simulink model "GS_model"  (R2018b)
settings: Solver=ode5  StartTime=0.0  StopTime=SimuStopTime  FixedStep=T_Simu  RelTol=1e-3
InitFcn:
  | Initial
undefined symbols (not defined in the file or in its folder): Aba10, Aba20, aeroCIP2006_S, aeroCIP2006_X, aeroCIP2006_Y, Agl0, Ass_kS, Ass_n1, Ass_n2, Ass_n3, Ass_n4, Ass_Noise, Ass_R, Ass_Resolution, Ass_TmOrder, AssA_Fix_Abs, AssB_Fix_Abs, AssC_Fix_Abs, AssD_Fix_Abs, AssE_Fix_Aps, AssF_Fix_Aps, C, c_max, c_min, Cd, CenterOfFigNX, CenterOfFigNY, CenterOfFigNZ, CenterOfFigP1, CenterOfFigP2, CenterOfFigPX, CenterOfFigPY, CenterOfFigPZ, Cmu, Crou, DEG2RAD, DiscIntNeverNeededParam, Eg_Dir, Eg_F, Eg_PrepareTime, Eg_r_L_L, Fw_Abf, Fw_Hmax, Fw_J, Fw_Spd0, Fw_Tmax, git_hash_BaseLine, git_hash_Project, Gnss_Noise_Pos, Gnss_Noise_Vel, Gnss_PropgationTime, GyroA_Fix_Abg, GyroA_Noise, GyroB_Fix_Abg, GyroB_Noise, GyroC_Fix_Abg, GyroC_Noise, GyroD_Fix_Abg, GyroD_Noise, h ... (+94)
libraries: simulink x308, sharedutil x46, aerolibutil x37, sharedtransform x31, vrlib x14, aerolibgravity2 x2
(part 13 of 20)

== system GS_model/Subsystem2/Subsystem/Sensor/StA&B&C&DModel1/StAMathModel3/Subsystem/Subsystem ==
  note: Qbs
  Sun_b : Inport
  Sunshine : Inport  Port=2
  Qsb_StAFix : Inport  Port=3
  SEA : Inport  Port=4
  EEA : Inport  Port=5
  Qob : Inport  Port=6
  Acos : Trigonometry  Operator=acos
  Acos1 : Trigonometry  Operator=acos
  Compare To Constant : simulink/Logic and Bit Operations/Compare To Constant  relop===  const=1  OutDataTypeStr=boolean
  Constant : Constant  Value=St_SightAxis
  Constant1 : Constant  Value=[0;0;1]
  Constant3 : Constant  Value=St_EarthAtomAgl
  Cos : Trigonometry  Operator=cos
  Cos1 : Trigonometry  Operator=cos
  Data Type Conversion : DataTypeConversion  OutDataTypeStr=double
  Logical Operator : Logic  AllPortsSameDT=off  OutDataTypeStr=boolean
  Logical Operator1 : Logic  Operator=OR  AllPortsSameDT=off  OutDataTypeStr=boolean
  Logical Operator2 : Logic  Operator=NOT  AllPortsSameDT=off  OutDataTypeStr=boolean
  MatrixMultiply{,1..4} (5 alike) : Product  Multiplication=Matrix(*)
  Mux : Mux  Inputs=2
  Quaternion Inverse : aerolibutil/Quaternion Inverse
  Quaternions to Direction Cosine Matrix : sharedtransform/Quaternions to  Direction Cosine Matrix  aMode=aMode
      settings: SourceProductBaseCode=AE,PW,MT,VE,VP
  Quaternions to Direction Cosine Matrix1 : sharedtransform/Quaternions to  Direction Cosine Matrix  aMode=aMode
      settings: SourceProductBaseCode=AE,PW,MT,VE,VP
  Relational Operator : RelationalOperator  OutDataTypeStr=boolean  RndMeth=Simplest
  Relational Operator1 : RelationalOperator  OutDataTypeStr=boolean  RndMeth=Simplest
  Sum : Sum  Inputs=|++
  Transpose : Math  Operator=transpose  SaturateOnIntegerOverflow=on
  Valid : Outport
  Agl_St&SunEarth : Outport  Port=2
  wires:
  Logical Operator1/1 -> Logical Operator2/1
  Data Type Conversion/1 -> Valid/1
  Logical Operator2/1 -> Data Type Conversion/1
  Mux/1 -> Agl_St&SunEarth/1
  MatrixMultiply/1 -> MatrixMultiply1/2
  Compare To Constant/1 -> Logical Operator/1
  MatrixMultiply1/1 -> Acos/1, Relational Operator/1
  Sum/1 -> Cos1/1
  Acos1/1 -> Mux/2
  Acos/1 -> Mux/1
  Relational Operator1/1 -> Logical Operator1/2
  EEA/1 -> Sum/1
  Sunshine/1 -> Compare To Constant/1
  MatrixMultiply4/1 -> Relational Operator1/1, Acos1/1
  Constant/1 -> Transpose/1
  Relational Operator/1 -> Logical Operator/2
  Quaternion Inverse/1 -> Quaternions to Direction Cosine Matrix/1
  Cos1/1 -> Relational Operator1/2
  MatrixMultiply2/1 -> MatrixMultiply3/2
  Constant1/1 -> MatrixMultiply2/2
  Sun_b/1 -> MatrixMultiply/2
  Quaternions to Direction Cosine Matrix/1 -> MatrixMultiply/1, MatrixMultiply3/1
  Qsb_StAFix/1 -> Quaternion Inverse/1
  MatrixMultiply3/1 -> MatrixMultiply4/2
  Qob/1 -> Quaternions to Direction Cosine Matrix1/1
  SEA/1 -> Cos/1
  Quaternions to Direction Cosine Matrix1/1 -> MatrixMultiply2/1
  Cos/1 -> Relational Operator/2
  Logical Operator/1 -> Logical Operator1/1
  Constant3/1 -> Sum/2
  Transpose/1 -> MatrixMultiply1/1, MatrixMultiply4/1

== system GS_model/Subsystem2/Subsystem/Sensor/StA&B&C&DModel1/StAMathModel3/Subsystem/Triggered Subsystem2 ==
  In1 : Inport
  Enable : EnablePort
  Out1 : Outport  InitialOutput=1
  wires:
  In1/1 -> Out1/1

== system GS_model/Subsystem2/EquipmentCmd/Fw1/Subsystem7/Subsystem1/FWDataSourceChoice/CmdModeChoice/422 ==
  In1 : Inport
  Action Port : ActionPort  ActionType=then
  Out1 : Outport
  wires:
  In1/1 -> Out1/1

== system GS_model/Subsystem2/EquipmentCmd/Fw1/Subsystem7/Subsystem1/FWDataSourceChoice/CmdModeChoice/FC ==
  In1 : Inport
  Action Port : ActionPort  ActionType=else
  Out1 : Outport
  wires:
  In1/1 -> Out1/1

== system GS_model/Subsystem2/EquipmentCmd/Fw1/Subsystem7/Subsystem1/FWDataSourceChoice/CmdModeChoice/UDP ==
  In1 : Inport
  Action Port : ActionPort  ActionType=elseif
  Out1 : Outport
  wires:
  In1/1 -> Out1/1

== system GS_model/Subsystem2/EquipmentCmd/Fw1/Subsystem7/Subsystem1/FWDataSourceChoice/CmdSpdChoice/422 ==
  In1 : Inport
  Action Port : ActionPort  ActionType=then
  Out1 : Outport
  wires:
  In1/1 -> Out1/1

== system GS_model/Subsystem2/EquipmentCmd/Fw1/Subsystem7/Subsystem1/FWDataSourceChoice/CmdSpdChoice/FC ==
  In1 : Inport
  Action Port : ActionPort  ActionType=else
  Out1 : Outport
  wires:
  In1/1 -> Out1/1

== system GS_model/Subsystem2/EquipmentCmd/Fw1/Subsystem7/Subsystem1/FWDataSourceChoice/CmdSpdChoice/UDP ==
  In1 : Inport
  Action Port : ActionPort  ActionType=elseif
  Out1 : Outport
  wires:
  In1/1 -> Out1/1

== system GS_model/Subsystem2/EquipmentCmd/Fw1/Subsystem7/Subsystem1/FWDataSourceChoice/CmdTChoice/422 ==
  In1 : Inport
  Action Port : ActionPort  ActionType=then
  Out1 : Outport
  wires:
  In1/1 -> Out1/1

== system GS_model/Subsystem2/EquipmentCmd/Fw1/Subsystem7/Subsystem1/FWDataSourceChoice/CmdTChoice/FC ==
  In1 : Inport
  Action Port : ActionPort  ActionType=else
  Out1 : Outport
  wires:
  In1/1 -> Out1/1

== system GS_model/Subsystem2/EquipmentCmd/Fw1/Subsystem7/Subsystem1/FWDataSourceChoice/CmdTChoice/UDP ==
  In1 : Inport
  Action Port : ActionPort  ActionType=elseif
  Out1 : Outport
  wires:
  In1/1 -> Out1/1

== system GS_model/Subsystem2/EquipmentCmd/Fw1/Subsystem7/Subsystem2/FWDataSourceChoice/CmdModeChoice/422 ==
  In1 : Inport
  Action Port : ActionPort  ActionType=then
  Out1 : Outport
  wires:
  In1/1 -> Out1/1

== system GS_model/Subsystem2/EquipmentCmd/Fw1/Subsystem7/Subsystem2/FWDataSourceChoice/CmdModeChoice/FC ==
  In1 : Inport
  Action Port : ActionPort  ActionType=else
  Out1 : Outport
  wires:
  In1/1 -> Out1/1

== system GS_model/Subsystem2/EquipmentCmd/Fw1/Subsystem7/Subsystem2/FWDataSourceChoice/CmdModeChoice/UDP ==
  In1 : Inport
  Action Port : ActionPort  ActionType=elseif
  Out1 : Outport
  wires:
  In1/1 -> Out1/1

== system GS_model/Subsystem2/EquipmentCmd/Fw1/Subsystem7/Subsystem2/FWDataSourceChoice/CmdSpdChoice/422 ==
  In1 : Inport
  Action Port : ActionPort  ActionType=then
  Out1 : Outport
  wires:
  In1/1 -> Out1/1

== system GS_model/Subsystem2/EquipmentCmd/Fw1/Subsystem7/Subsystem2/FWDataSourceChoice/CmdSpdChoice/FC ==
  In1 : Inport
  Action Port : ActionPort  ActionType=else
  Out1 : Outport
  wires:
  In1/1 -> Out1/1

== system GS_model/Subsystem2/EquipmentCmd/Fw1/Subsystem7/Subsystem2/FWDataSourceChoice/CmdSpdChoice/UDP ==
  In1 : Inport
  Action Port : ActionPort  ActionType=elseif
  Out1 : Outport
  wires:
  In1/1 -> Out1/1

== system GS_model/Subsystem2/EquipmentCmd/Fw1/Subsystem7/Subsystem2/FWDataSourceChoice/CmdTChoice/422 ==
  In1 : Inport
  Action Port : ActionPort  ActionType=then
  Out1 : Outport
  wires:
  In1/1 -> Out1/1

== system GS_model/Subsystem2/EquipmentCmd/Fw1/Subsystem7/Subsystem2/FWDataSourceChoice/CmdTChoice/FC ==
  In1 : Inport
  Action Port : ActionPort  ActionType=else
  Out1 : Outport
  wires:
  In1/1 -> Out1/1

== system GS_model/Subsystem2/EquipmentCmd/Fw1/Subsystem7/Subsystem2/FWDataSourceChoice/CmdTChoice/UDP ==
  In1 : Inport
  Action Port : ActionPort  ActionType=elseif
  Out1 : Outport
  wires:
  In1/1 -> Out1/1

== system GS_model/Subsystem2/EquipmentCmd/Fw1/Subsystem7/Subsystem3/FWDataSourceChoice/CmdModeChoice/422 ==
  In1 : Inport
  Action Port : ActionPort  ActionType=then
  Out1 : Outport
  wires:
  In1/1 -> Out1/1

== system GS_model/Subsystem2/EquipmentCmd/Fw1/Subsystem7/Subsystem3/FWDataSourceChoice/CmdModeChoice/FC ==
  In1 : Inport
  Action Port : ActionPort  ActionType=else
  Out1 : Outport
  wires:
  In1/1 -> Out1/1

== system GS_model/Subsystem2/EquipmentCmd/Fw1/Subsystem7/Subsystem3/FWDataSourceChoice/CmdModeChoice/UDP ==
  In1 : Inport
  Action Port : ActionPort  ActionType=elseif
  Out1 : Outport
  wires:
  In1/1 -> Out1/1

== system GS_model/Subsystem2/EquipmentCmd/Fw1/Subsystem7/Subsystem3/FWDataSourceChoice/CmdSpdChoice/422 ==
  In1 : Inport
  Action Port : ActionPort  ActionType=then
  Out1 : Outport
  wires:
  In1/1 -> Out1/1

== system GS_model/Subsystem2/EquipmentCmd/Fw1/Subsystem7/Subsystem3/FWDataSourceChoice/CmdSpdChoice/FC ==
  In1 : Inport
  Action Port : ActionPort  ActionType=else
  Out1 : Outport
  wires:
  In1/1 -> Out1/1

== system GS_model/Subsystem2/EquipmentCmd/Fw1/Subsystem7/Subsystem3/FWDataSourceChoice/CmdSpdChoice/UDP ==
  In1 : Inport
  Action Port : ActionPort  ActionType=elseif
  Out1 : Outport
  wires:
  In1/1 -> Out1/1

== system GS_model/Subsystem2/EquipmentCmd/Fw1/Subsystem7/Subsystem3/FWDataSourceChoice/CmdTChoice/422 ==
  In1 : Inport
  Action Port : ActionPort  ActionType=then
  Out1 : Outport
  wires:
  In1/1 -> Out1/1

== system GS_model/Subsystem2/EquipmentCmd/Fw1/Subsystem7/Subsystem3/FWDataSourceChoice/CmdTChoice/FC ==
  In1 : Inport
  Action Port : ActionPort  ActionType=else
  Out1 : Outport
  wires:
  In1/1 -> Out1/1

== system GS_model/Subsystem2/EquipmentCmd/Fw1/Subsystem7/Subsystem3/FWDataSourceChoice/CmdTChoice/UDP ==
  In1 : Inport
  Action Port : ActionPort  ActionType=elseif
  Out1 : Outport
  wires:
  In1/1 -> Out1/1

== system GS_model/Subsystem2/EquipmentCmd/Fw1/Subsystem7/Subsystem4/FWDataSourceChoice/CmdModeChoice/422 ==
  In1 : Inport
  Action Port : ActionPort  ActionType=then
  Out1 : Outport
  wires:
  In1/1 -> Out1/1

== system GS_model/Subsystem2/EquipmentCmd/Fw1/Subsystem7/Subsystem4/FWDataSourceChoice/CmdModeChoice/FC ==
  In1 : Inport
  Action Port : ActionPort  ActionType=else
  Out1 : Outport
  wires:
  In1/1 -> Out1/1

== system GS_model/Subsystem2/EquipmentCmd/Fw1/Subsystem7/Subsystem4/FWDataSourceChoice/CmdModeChoice/UDP ==
  In1 : Inport
  Action Port : ActionPort  ActionType=elseif
  Out1 : Outport
  wires:
  In1/1 -> Out1/1

== system GS_model/Subsystem2/EquipmentCmd/Fw1/Subsystem7/Subsystem4/FWDataSourceChoice/CmdSpdChoice/422 ==
  In1 : Inport
  Action Port : ActionPort  ActionType=then
  Out1 : Outport
  wires:
  In1/1 -> Out1/1

== system GS_model/Subsystem2/EquipmentCmd/Fw1/Subsystem7/Subsystem4/FWDataSourceChoice/CmdSpdChoice/FC ==
  In1 : Inport
  Action Port : ActionPort  ActionType=else
  Out1 : Outport
  wires:
  In1/1 -> Out1/1

== system GS_model/Subsystem2/EquipmentCmd/Fw1/Subsystem7/Subsystem4/FWDataSourceChoice/CmdSpdChoice/UDP ==
  In1 : Inport
  Action Port : ActionPort  ActionType=elseif
  Out1 : Outport
  wires:
  In1/1 -> Out1/1

== system GS_model/Subsystem2/EquipmentCmd/Fw1/Subsystem7/Subsystem4/FWDataSourceChoice/CmdTChoice/422 ==
  In1 : Inport
  Action Port : ActionPort  ActionType=then
  Out1 : Outport
  wires:
  In1/1 -> Out1/1

== system GS_model/Subsystem2/EquipmentCmd/Fw1/Subsystem7/Subsystem4/FWDataSourceChoice/CmdTChoice/FC ==
  In1 : Inport
  Action Port : ActionPort  ActionType=else
  Out1 : Outport
  wires:
  In1/1 -> Out1/1

== system GS_model/Subsystem2/EquipmentCmd/Fw1/Subsystem7/Subsystem4/FWDataSourceChoice/CmdTChoice/UDP ==
  In1 : Inport
  Action Port : ActionPort  ActionType=elseif
  Out1 : Outport
  wires:
  In1/1 -> Out1/1

== system GS_model/Subsystem2/EquipmentCmd/Fw1/Subsystem7/Subsystem5/FWDataSourceChoice/CmdModeChoice/422 ==
  In1 : Inport
  Action Port : ActionPort  ActionType=then
  Out1 : Outport
  wires:
  In1/1 -> Out1/1

== system GS_model/Subsystem2/EquipmentCmd/Fw1/Subsystem7/Subsystem5/FWDataSourceChoice/CmdModeChoice/FC ==
  In1 : Inport
  Action Port : ActionPort  ActionType=else
  Out1 : Outport
  wires:
  In1/1 -> Out1/1

== system GS_model/Subsystem2/EquipmentCmd/Fw1/Subsystem7/Subsystem5/FWDataSourceChoice/CmdModeChoice/UDP ==
  In1 : Inport
  Action Port : ActionPort  ActionType=elseif
  Out1 : Outport
  wires:
  In1/1 -> Out1/1

== system GS_model/Subsystem2/EquipmentCmd/Fw1/Subsystem7/Subsystem5/FWDataSourceChoice/CmdSpdChoice/422 ==
  In1 : Inport
  Action Port : ActionPort  ActionType=then
  Out1 : Outport
  wires:
  In1/1 -> Out1/1

== system GS_model/Subsystem2/EquipmentCmd/Fw1/Subsystem7/Subsystem5/FWDataSourceChoice/CmdSpdChoice/FC ==
  In1 : Inport
  Action Port : ActionPort  ActionType=else
  Out1 : Outport
  wires:
  In1/1 -> Out1/1

== system GS_model/Subsystem2/EquipmentCmd/Fw1/Subsystem7/Subsystem5/FWDataSourceChoice/CmdSpdChoice/UDP ==
  In1 : Inport
  Action Port : ActionPort  ActionType=elseif
  Out1 : Outport
  wires:
  In1/1 -> Out1/1

== system GS_model/Subsystem2/EquipmentCmd/Fw1/Subsystem7/Subsystem5/FWDataSourceChoice/CmdTChoice/422 ==
  In1 : Inport
  Action Port : ActionPort  ActionType=then
  Out1 : Outport
  wires:
  In1/1 -> Out1/1

== system GS_model/Subsystem2/EquipmentCmd/Fw1/Subsystem7/Subsystem5/FWDataSourceChoice/CmdTChoice/FC ==
  In1 : Inport
  Action Port : ActionPort  ActionType=else
  Out1 : Outport
  wires:
  In1/1 -> Out1/1

== system GS_model/Subsystem2/EquipmentCmd/Fw1/Subsystem7/Subsystem5/FWDataSourceChoice/CmdTChoice/UDP ==
  In1 : Inport
  Action Port : ActionPort  ActionType=elseif
  Out1 : Outport
  wires:
  In1/1 -> Out1/1

== system GS_model/Subsystem2/EquipmentCmd/Fw1/Subsystem7/Subsystem6/FWDataSourceChoice/CmdModeChoice/422 ==
  In1 : Inport
  Action Port : ActionPort  ActionType=then
  Out1 : Outport
  wires:
  In1/1 -> Out1/1

== system GS_model/Subsystem2/EquipmentCmd/Fw1/Subsystem7/Subsystem6/FWDataSourceChoice/CmdModeChoice/FC ==
  In1 : Inport
  Action Port : ActionPort  ActionType=else
  Out1 : Outport
  wires:
  In1/1 -> Out1/1

== system GS_model/Subsystem2/EquipmentCmd/Fw1/Subsystem7/Subsystem6/FWDataSourceChoice/CmdModeChoice/UDP ==
  In1 : Inport
  Action Port : ActionPort  ActionType=elseif
  Out1 : Outport
  wires:
  In1/1 -> Out1/1

== system GS_model/Subsystem2/EquipmentCmd/Fw1/Subsystem7/Subsystem6/FWDataSourceChoice/CmdSpdChoice/422 ==
  In1 : Inport
  Action Port : ActionPort  ActionType=then
  Out1 : Outport
  wires:
  In1/1 -> Out1/1

== system GS_model/Subsystem2/EquipmentCmd/Fw1/Subsystem7/Subsystem6/FWDataSourceChoice/CmdSpdChoice/FC ==
  In1 : Inport
  Action Port : ActionPort  ActionType=else
  Out1 : Outport
  wires:
  In1/1 -> Out1/1

== system GS_model/Subsystem2/EquipmentCmd/Fw1/Subsystem7/Subsystem6/FWDataSourceChoice/CmdSpdChoice/UDP ==
  In1 : Inport
  Action Port : ActionPort  ActionType=elseif
  Out1 : Outport
  wires:
  In1/1 -> Out1/1

== system GS_model/Subsystem2/EquipmentCmd/Fw1/Subsystem7/Subsystem6/FWDataSourceChoice/CmdTChoice/422 ==
  In1 : Inport
  Action Port : ActionPort  ActionType=then
  Out1 : Outport
  wires:
  In1/1 -> Out1/1

== system GS_model/Subsystem2/EquipmentCmd/Fw1/Subsystem7/Subsystem6/FWDataSourceChoice/CmdTChoice/FC ==
  In1 : Inport
  Action Port : ActionPort  ActionType=else
  Out1 : Outport
  wires:
  In1/1 -> Out1/1

== system GS_model/Subsystem2/EquipmentCmd/Fw1/Subsystem7/Subsystem6/FWDataSourceChoice/CmdTChoice/UDP ==
  In1 : Inport
  Action Port : ActionPort  ActionType=elseif
  Out1 : Outport
  wires:
  In1/1 -> Out1/1

== system GS_model/Subsystem2/Subsystem/Actuator/FlyWheel/FwAModel1/FWDataSourceChoice/DelayModel/delay1 ==
  In1 : Inport
  In2 : Inport  Port=2
  Delay : Delay  DelayLength=floor(T_Ctrl/T_Simu)
  Delay1 : Delay  DelayLength=2*floor(T_Ctrl/T_Simu)
  Delay2 : Delay  DelayLength=3*floor(T_Ctrl/T_Simu)
  Delay3 : Delay  DelayLength=4*floor(T_Ctrl/T_Simu)
  Multiport Switch : MultiPortSwitch  Inputs=5  SaturateOnIntegerOverflow=on
  Out1 : Outport
  wires:
  Delay1/1 -> Multiport Switch/4
  Delay2/1 -> Multiport Switch/5
  Delay3/1 -> Multiport Switch/6
  In1/1 -> Multiport Switch/1
  Multiport Switch/1 -> Out1/1
  In2/1 -> Multiport Switch/2, Delay1/1, Delay2/1, Delay3/1, Delay/1
  Delay/1 -> Multiport Switch/3

== system GS_model/Subsystem2/Subsystem/Actuator/FlyWheel/FwAModel1/FWDataSourceChoice/DelayModel/delay2 ==
  In1 : Inport
  In2 : Inport  Port=2
  Delay : Delay  DelayLength=floor(T_Ctrl/T_Simu)
  Delay1 : Delay  DelayLength=2*floor(T_Ctrl/T_Simu)
  Delay2 : Delay  DelayLength=3*floor(T_Ctrl/T_Simu)
  Delay3 : Delay  DelayLength=4*floor(T_Ctrl/T_Simu)
  Multiport Switch : MultiPortSwitch  Inputs=5  SaturateOnIntegerOverflow=on
  Out1 : Outport
  wires:
  Delay/1 -> Multiport Switch/3
  In2/1 -> Delay/1, Delay3/1, Delay2/1, Delay1/1, Multiport Switch/2
  Multiport Switch/1 -> Out1/1
  In1/1 -> Multiport Switch/1
  Delay3/1 -> Multiport Switch/6
  Delay2/1 -> Multiport Switch/5
  Delay1/1 -> Multiport Switch/4

== system GS_model/Subsystem2/Subsystem/Actuator/FlyWheel/FwAModel1/FWDataSourceChoice/DelayModel/delay3 ==
  In1 : Inport
  In2 : Inport  Port=2
  Delay : Delay  DelayLength=floor(T_Ctrl/T_Simu)
  Delay1 : Delay  DelayLength=2*floor(T_Ctrl/T_Simu)
  Delay2 : Delay  DelayLength=3*floor(T_Ctrl/T_Simu)
  Delay3 : Delay  DelayLength=4*floor(T_Ctrl/T_Simu)
  Multiport Switch : MultiPortSwitch  Inputs=5  SaturateOnIntegerOverflow=on
  Out1 : Outport
  wires:
  Delay1/1 -> Multiport Switch/4
  Delay2/1 -> Multiport Switch/5
  Delay3/1 -> Multiport Switch/6
  In1/1 -> Multiport Switch/1
  Multiport Switch/1 -> Out1/1
  In2/1 -> Multiport Switch/2, Delay1/1, Delay2/1, Delay3/1, Delay/1
  Delay/1 -> Multiport Switch/3

== system GS_model/Subsystem2/Subsystem/Actuator/FlyWheel/FwAModel1/FWMath&ErrModel/Subsystem1/If Action Subsystem ==
  In1 : Inport
  Action Port : ActionPort  ActionType=then
  Out1 : Outport
  wires:
  In1/1 -> Out1/1

== system GS_model/Subsystem2/Subsystem/Actuator/FlyWheel/FwAModel1/FWMath&ErrModel/Subsystem1/If Action Subsystem1 ==
  In1 : Inport
  Action Port : ActionPort  ActionType=else
  Out1 : Outport
  wires:
  In1/1 -> Out1/1

== system GS_model/Subsystem2/Subsystem/Actuator/FlyWheel/FwAModel1/FWMath&ErrModel/Subsystem1/Triggered Subsystem1 ==
  In1 : Inport
  Enable : EnablePort
  Out1 : Outport  InitialOutput=0
  wires:
  In1/1 -> Out1/1

== system GS_model/Subsystem2/Subsystem/Actuator/FlyWheel/FwAModel1/FWMath&ErrModel/Subsystem1/Triggered Subsystem2 ==
  In1 : Inport
  Enable : EnablePort
  Out1 : Outport  InitialOutput=0
  wires:
  In1/1 -> Out1/1

== system GS_model/Subsystem2/Subsystem/Actuator/FlyWheel/FwAModel1/FWMath&ErrModel/Subsystem2/If Action Subsystem ==
  In1 : Inport
  Action Port : ActionPort  ActionType=then
  Out1 : Outport
  wires:
  In1/1 -> Out1/1

== system GS_model/Subsystem2/Subsystem/Actuator/FlyWheel/FwAModel1/FWMath&ErrModel/Subsystem2/If Action Subsystem1 ==
  In1 : Inport
  Action Port : ActionPort  ActionType=else
  Out1 : Outport
  wires:
  In1/1 -> Out1/1

== system GS_model/Subsystem2/Subsystem/Actuator/FlyWheel/FwAModel1/FWMath&ErrModel/Subsystem2/Triggered Subsystem1 ==
  In1 : Inport
  Enable : EnablePort
  Out1 : Outport  InitialOutput=0
  wires:
  In1/1 -> Out1/1

== system GS_model/Subsystem2/Subsystem/Actuator/FlyWheel/FwAModel1/FWMath&ErrModel/Subsystem2/Triggered Subsystem2 ==
  In1 : Inport
  Enable : EnablePort
  Out1 : Outport  InitialOutput=0
  wires:
  In1/1 -> Out1/1

== system GS_model/Subsystem2/Subsystem/Actuator/FlyWheel/FwAModel1/FWMath&ErrModel/Subsystem4/If Action Subsystem ==
  In1 : Inport
  Action Port : ActionPort  ActionType=then
  Out1 : Outport
  wires:
  In1/1 -> Out1/1

== system GS_model/Subsystem2/Subsystem/Actuator/FlyWheel/FwAModel1/FWMath&ErrModel/Subsystem4/If Action Subsystem1 ==
  In1 : Inport
  Action Port : ActionPort  ActionType=else
  Out1 : Outport
  wires:
  In1/1 -> Out1/1

== system GS_model/Subsystem2/Subsystem/Actuator/FlyWheel/FwAModel1/FWMath&ErrModel/Subsystem4/Triggered Subsystem1 ==
  In1 : Inport
  Enable : EnablePort
  Out1 : Outport  InitialOutput=0
  wires:
  In1/1 -> Out1/1

== system GS_model/Subsystem2/Subsystem/Actuator/FlyWheel/FwAModel2/FWDataSourceChoice/DelayModel/delay1 ==
  In1 : Inport
  In2 : Inport  Port=2
  Delay : Delay  DelayLength=floor(T_Ctrl/T_Simu)
  Delay1 : Delay  DelayLength=2*floor(T_Ctrl/T_Simu)
  Delay2 : Delay  DelayLength=3*floor(T_Ctrl/T_Simu)
  Delay3 : Delay  DelayLength=4*floor(T_Ctrl/T_Simu)
  Multiport Switch : MultiPortSwitch  Inputs=5  SaturateOnIntegerOverflow=on
  Out1 : Outport
  wires:
  Delay/1 -> Multiport Switch/3
  In2/1 -> Delay/1, Delay3/1, Delay2/1, Delay1/1, Multiport Switch/2
  Multiport Switch/1 -> Out1/1
  In1/1 -> Multiport Switch/1
  Delay3/1 -> Multiport Switch/6
  Delay2/1 -> Multiport Switch/5
  Delay1/1 -> Multiport Switch/4

== system GS_model/Subsystem2/Subsystem/Actuator/FlyWheel/FwAModel2/FWDataSourceChoice/DelayModel/delay2 ==
  In1 : Inport
  In2 : Inport  Port=2
  Delay : Delay  DelayLength=floor(T_Ctrl/T_Simu)
  Delay1 : Delay  DelayLength=2*floor(T_Ctrl/T_Simu)
  Delay2 : Delay  DelayLength=3*floor(T_Ctrl/T_Simu)
  Delay3 : Delay  DelayLength=4*floor(T_Ctrl/T_Simu)
  Multiport Switch : MultiPortSwitch  Inputs=5  SaturateOnIntegerOverflow=on
  Out1 : Outport
  wires:
  Delay1/1 -> Multiport Switch/4
  Delay2/1 -> Multiport Switch/5
  Delay3/1 -> Multiport Switch/6
  In1/1 -> Multiport Switch/1
  Multiport Switch/1 -> Out1/1
  In2/1 -> Multiport Switch/2, Delay1/1, Delay2/1, Delay3/1, Delay/1
  Delay/1 -> Multiport Switch/3

== system GS_model/Subsystem2/Subsystem/Actuator/FlyWheel/FwAModel2/FWDataSourceChoice/DelayModel/delay3 ==
  In1 : Inport
  In2 : Inport  Port=2
  Delay : Delay  DelayLength=floor(T_Ctrl/T_Simu)
  Delay1 : Delay  DelayLength=2*floor(T_Ctrl/T_Simu)
  Delay2 : Delay  DelayLength=3*floor(T_Ctrl/T_Simu)
  Delay3 : Delay  DelayLength=4*floor(T_Ctrl/T_Simu)
  Multiport Switch : MultiPortSwitch  Inputs=5  SaturateOnIntegerOverflow=on
  Out1 : Outport
  wires:
  Delay/1 -> Multiport Switch/3
  In2/1 -> Delay/1, Delay3/1, Delay2/1, Delay1/1, Multiport Switch/2
  Multiport Switch/1 -> Out1/1
  In1/1 -> Multiport Switch/1
  Delay3/1 -> Multiport Switch/6
  Delay2/1 -> Multiport Switch/5
  Delay1/1 -> Multiport Switch/4

== system GS_model/Subsystem2/Subsystem/Actuator/FlyWheel/FwAModel2/FWMath&ErrModel/Subsystem1/If Action Subsystem ==
  In1 : Inport
  Action Port : ActionPort  ActionType=then
  Out1 : Outport
  wires:
  In1/1 -> Out1/1

== system GS_model/Subsystem2/Subsystem/Actuator/FlyWheel/FwAModel2/FWMath&ErrModel/Subsystem1/If Action Subsystem1 ==
  In1 : Inport
  Action Port : ActionPort  ActionType=else
  Out1 : Outport
  wires:
  In1/1 -> Out1/1

== system GS_model/Subsystem2/Subsystem/Actuator/FlyWheel/FwAModel2/FWMath&ErrModel/Subsystem1/Triggered Subsystem1 ==
  In1 : Inport
  Enable : EnablePort
  Out1 : Outport  InitialOutput=0
  wires:
  In1/1 -> Out1/1

== system GS_model/Subsystem2/Subsystem/Actuator/FlyWheel/FwAModel2/FWMath&ErrModel/Subsystem1/Triggered Subsystem2 ==
  In1 : Inport
  Enable : EnablePort
  Out1 : Outport  InitialOutput=0
  wires:
  In1/1 -> Out1/1

== system GS_model/Subsystem2/Subsystem/Actuator/FlyWheel/FwAModel2/FWMath&ErrModel/Subsystem2/If Action Subsystem ==
  In1 : Inport
  Action Port : ActionPort  ActionType=then
  Out1 : Outport
  wires:
  In1/1 -> Out1/1

== system GS_model/Subsystem2/Subsystem/Actuator/FlyWheel/FwAModel2/FWMath&ErrModel/Subsystem2/If Action Subsystem1 ==
  In1 : Inport
  Action Port : ActionPort  ActionType=else
  Out1 : Outport
  wires:
  In1/1 -> Out1/1

== system GS_model/Subsystem2/Subsystem/Actuator/FlyWheel/FwAModel2/FWMath&ErrModel/Subsystem2/Triggered Subsystem1 ==
  In1 : Inport
  Enable : EnablePort
  Out1 : Outport  InitialOutput=0
  wires:
  In1/1 -> Out1/1

== system GS_model/Subsystem2/Subsystem/Actuator/FlyWheel/FwAModel2/FWMath&ErrModel/Subsystem2/Triggered Subsystem2 ==
  In1 : Inport
  Enable : EnablePort
  Out1 : Outport  InitialOutput=0
  wires:
  In1/1 -> Out1/1

== system GS_model/Subsystem2/Subsystem/Actuator/FlyWheel/FwAModel2/FWMath&ErrModel/Subsystem4/If Action Subsystem ==
  In1 : Inport
  Action Port : ActionPort  ActionType=then
  Out1 : Outport
  wires:
  In1/1 -> Out1/1

== system GS_model/Subsystem2/Subsystem/Actuator/FlyWheel/FwAModel2/FWMath&ErrModel/Subsystem4/If Action Subsystem1 ==
  In1 : Inport
  Action Port : ActionPort  ActionType=else
  Out1 : Outport
  wires:
  In1/1 -> Out1/1

== system GS_model/Subsystem2/Subsystem/Actuator/FlyWheel/FwAModel2/FWMath&ErrModel/Subsystem4/Triggered Subsystem1 ==
  In1 : Inport
  Enable : EnablePort
  Out1 : Outport  InitialOutput=0
  wires:
  In1/1 -> Out1/1

== system GS_model/Subsystem2/Subsystem/Actuator/FlyWheel/FwAModel3/FWDataSourceChoice/DelayModel/delay1 ==
  In1 : Inport
  In2 : Inport  Port=2
  Delay : Delay  DelayLength=floor(T_Ctrl/T_Simu)
  Delay1 : Delay  DelayLength=2*floor(T_Ctrl/T_Simu)
  Delay2 : Delay  DelayLength=3*floor(T_Ctrl/T_Simu)
  Delay3 : Delay  DelayLength=4*floor(T_Ctrl/T_Simu)
  Multiport Switch : MultiPortSwitch  Inputs=5  SaturateOnIntegerOverflow=on
  Out1 : Outport
  wires:
  Delay1/1 -> Multiport Switch/4
  Delay2/1 -> Multiport Switch/5
  Delay3/1 -> Multiport Switch/6
  In1/1 -> Multiport Switch/1
  Multiport Switch/1 -> Out1/1
  In2/1 -> Multiport Switch/2, Delay1/1, Delay2/1, Delay3/1, Delay/1
  Delay/1 -> Multiport Switch/3

== system GS_model/Subsystem2/Subsystem/Actuator/FlyWheel/FwAModel3/FWDataSourceChoice/DelayModel/delay2 ==
  In1 : Inport
  In2 : Inport  Port=2
  Delay : Delay  DelayLength=floor(T_Ctrl/T_Simu)
  Delay1 : Delay  DelayLength=2*floor(T_Ctrl/T_Simu)
  Delay2 : Delay  DelayLength=3*floor(T_Ctrl/T_Simu)
  Delay3 : Delay  DelayLength=4*floor(T_Ctrl/T_Simu)
  Multiport Switch : MultiPortSwitch  Inputs=5  SaturateOnIntegerOverflow=on
  Out1 : Outport
  wires:
  Delay/1 -> Multiport Switch/3
  In2/1 -> Delay/1, Delay3/1, Delay2/1, Delay1/1, Multiport Switch/2
  Multiport Switch/1 -> Out1/1
  In1/1 -> Multiport Switch/1
  Delay3/1 -> Multiport Switch/6
  Delay2/1 -> Multiport Switch/5
  Delay1/1 -> Multiport Switch/4

== system GS_model/Subsystem2/Subsystem/Actuator/FlyWheel/FwAModel3/FWDataSourceChoice/DelayModel/delay3 ==
  In1 : Inport
  In2 : Inport  Port=2
  Delay : Delay  DelayLength=floor(T_Ctrl/T_Simu)
  Delay1 : Delay  DelayLength=2*floor(T_Ctrl/T_Simu)
  Delay2 : Delay  DelayLength=3*floor(T_Ctrl/T_Simu)
  Delay3 : Delay  DelayLength=4*floor(T_Ctrl/T_Simu)
  Multiport Switch : MultiPortSwitch  Inputs=5  SaturateOnIntegerOverflow=on
  Out1 : Outport
  wires:
  Delay1/1 -> Multiport Switch/4
  Delay2/1 -> Multiport Switch/5
  Delay3/1 -> Multiport Switch/6
  In1/1 -> Multiport Switch/1
  Multiport Switch/1 -> Out1/1
  In2/1 -> Multiport Switch/2, Delay1/1, Delay2/1, Delay3/1, Delay/1
  Delay/1 -> Multiport Switch/3

== system GS_model/Subsystem2/Subsystem/Actuator/FlyWheel/FwAModel3/FWMath&ErrModel/Subsystem1/If Action Subsystem ==
  In1 : Inport
  Action Port : ActionPort  ActionType=then
  Out1 : Outport
  wires:
  In1/1 -> Out1/1

== system GS_model/Subsystem2/Subsystem/Actuator/FlyWheel/FwAModel3/FWMath&ErrModel/Subsystem1/If Action Subsystem1 ==
  In1 : Inport
  Action Port : ActionPort  ActionType=else
  Out1 : Outport
  wires:
  In1/1 -> Out1/1

== system GS_model/Subsystem2/Subsystem/Actuator/FlyWheel/FwAModel3/FWMath&ErrModel/Subsystem1/Triggered Subsystem1 ==
  In1 : Inport
  Enable : EnablePort
  Out1 : Outport  InitialOutput=0
  wires:
  In1/1 -> Out1/1

== system GS_model/Subsystem2/Subsystem/Actuator/FlyWheel/FwAModel3/FWMath&ErrModel/Subsystem1/Triggered Subsystem2 ==
  In1 : Inport
  Enable : EnablePort
  Out1 : Outport  InitialOutput=0
  wires:
  In1/1 -> Out1/1

== system GS_model/Subsystem2/Subsystem/Actuator/FlyWheel/FwAModel3/FWMath&ErrModel/Subsystem2/If Action Subsystem ==
  In1 : Inport
  Action Port : ActionPort  ActionType=then
  Out1 : Outport
  wires:
  In1/1 -> Out1/1

== system GS_model/Subsystem2/Subsystem/Actuator/FlyWheel/FwAModel3/FWMath&ErrModel/Subsystem2/If Action Subsystem1 ==
  In1 : Inport
  Action Port : ActionPort  ActionType=else
  Out1 : Outport
  wires:
  In1/1 -> Out1/1

== system GS_model/Subsystem2/Subsystem/Actuator/FlyWheel/FwAModel3/FWMath&ErrModel/Subsystem2/Triggered Subsystem1 ==
  In1 : Inport
  Enable : EnablePort
  Out1 : Outport  InitialOutput=0
  wires:
  In1/1 -> Out1/1

== system GS_model/Subsystem2/Subsystem/Actuator/FlyWheel/FwAModel3/FWMath&ErrModel/Subsystem2/Triggered Subsystem2 ==
  In1 : Inport
  Enable : EnablePort
  Out1 : Outport  InitialOutput=0
  wires:
  In1/1 -> Out1/1

== system GS_model/Subsystem2/Subsystem/Actuator/FlyWheel/FwAModel3/FWMath&ErrModel/Subsystem4/If Action Subsystem ==
  In1 : Inport
  Action Port : ActionPort  ActionType=then
  Out1 : Outport
  wires:
  In1/1 -> Out1/1

== system GS_model/Subsystem2/Subsystem/Actuator/FlyWheel/FwAModel3/FWMath&ErrModel/Subsystem4/If Action Subsystem1 ==
  In1 : Inport
  Action Port : ActionPort  ActionType=else
  Out1 : Outport
  wires:
  In1/1 -> Out1/1

== system GS_model/Subsystem2/Subsystem/Actuator/FlyWheel/FwAModel3/FWMath&ErrModel/Subsystem4/Triggered Subsystem1 ==
  In1 : Inport
  Enable : EnablePort
  Out1 : Outport  InitialOutput=0
  wires:
  In1/1 -> Out1/1

== system GS_model/Subsystem2/Subsystem/Actuator/FlyWheel/FwAModel4/FWDataSourceChoice/DelayModel/delay1 ==
  In1 : Inport
  In2 : Inport  Port=2
  Delay : Delay  DelayLength=floor(T_Ctrl/T_Simu)
  Delay1 : Delay  DelayLength=2*floor(T_Ctrl/T_Simu)
  Delay2 : Delay  DelayLength=3*floor(T_Ctrl/T_Simu)
  Delay3 : Delay  DelayLength=4*floor(T_Ctrl/T_Simu)
  Multiport Switch : MultiPortSwitch  Inputs=5  SaturateOnIntegerOverflow=on
  Out1 : Outport
  wires:
  Delay/1 -> Multiport Switch/3
  In2/1 -> Delay/1, Delay3/1, Delay2/1, Delay1/1, Multiport Switch/2
  Multiport Switch/1 -> Out1/1
  In1/1 -> Multiport Switch/1
  Delay3/1 -> Multiport Switch/6
  Delay2/1 -> Multiport Switch/5
  Delay1/1 -> Multiport Switch/4

== system GS_model/Subsystem2/Subsystem/Actuator/FlyWheel/FwAModel4/FWDataSourceChoice/DelayModel/delay2 ==
  In1 : Inport
  In2 : Inport  Port=2
  Delay : Delay  DelayLength=floor(T_Ctrl/T_Simu)
  Delay1 : Delay  DelayLength=2*floor(T_Ctrl/T_Simu)
  Delay2 : Delay  DelayLength=3*floor(T_Ctrl/T_Simu)
  Delay3 : Delay  DelayLength=4*floor(T_Ctrl/T_Simu)
  Multiport Switch : MultiPortSwitch  Inputs=5  SaturateOnIntegerOverflow=on
  Out1 : Outport
  wires:
  Delay1/1 -> Multiport Switch/4
  Delay2/1 -> Multiport Switch/5
  Delay3/1 -> Multiport Switch/6
  In1/1 -> Multiport Switch/1
  Multiport Switch/1 -> Out1/1
  In2/1 -> Multiport Switch/2, Delay1/1, Delay2/1, Delay3/1, Delay/1
  Delay/1 -> Multiport Switch/3

== system GS_model/Subsystem2/Subsystem/Actuator/FlyWheel/FwAModel4/FWDataSourceChoice/DelayModel/delay3 ==
  In1 : Inport
  In2 : Inport  Port=2
  Delay : Delay  DelayLength=floor(T_Ctrl/T_Simu)
  Delay1 : Delay  DelayLength=2*floor(T_Ctrl/T_Simu)
  Delay2 : Delay  DelayLength=3*floor(T_Ctrl/T_Simu)
  Delay3 : Delay  DelayLength=4*floor(T_Ctrl/T_Simu)
  Multiport Switch : MultiPortSwitch  Inputs=5  SaturateOnIntegerOverflow=on
  Out1 : Outport
  wires:
  Delay/1 -> Multiport Switch/3
  In2/1 -> Delay/1, Delay3/1, Delay2/1, Delay1/1, Multiport Switch/2
  Multiport Switch/1 -> Out1/1
  In1/1 -> Multiport Switch/1
  Delay3/1 -> Multiport Switch/6
  Delay2/1 -> Multiport Switch/5
  Delay1/1 -> Multiport Switch/4

== system GS_model/Subsystem2/Subsystem/Actuator/FlyWheel/FwAModel4/FWMath&ErrModel/Subsystem1/If Action Subsystem ==
  In1 : Inport
  Action Port : ActionPort  ActionType=then
  Out1 : Outport
  wires:
  In1/1 -> Out1/1

== system GS_model/Subsystem2/Subsystem/Actuator/FlyWheel/FwAModel4/FWMath&ErrModel/Subsystem1/If Action Subsystem1 ==
  In1 : Inport
  Action Port : ActionPort  ActionType=else
  Out1 : Outport
  wires:
  In1/1 -> Out1/1

== system GS_model/Subsystem2/Subsystem/Actuator/FlyWheel/FwAModel4/FWMath&ErrModel/Subsystem1/Triggered Subsystem1 ==
  In1 : Inport
  Enable : EnablePort
  Out1 : Outport  InitialOutput=0
  wires:
  In1/1 -> Out1/1

== system GS_model/Subsystem2/Subsystem/Actuator/FlyWheel/FwAModel4/FWMath&ErrModel/Subsystem1/Triggered Subsystem2 ==
  In1 : Inport
  Enable : EnablePort
  Out1 : Outport  InitialOutput=0
  wires:
  In1/1 -> Out1/1

== system GS_model/Subsystem2/Subsystem/Actuator/FlyWheel/FwAModel4/FWMath&ErrModel/Subsystem2/If Action Subsystem ==
  In1 : Inport
  Action Port : ActionPort  ActionType=then
  Out1 : Outport
  wires:
  In1/1 -> Out1/1

== system GS_model/Subsystem2/Subsystem/Actuator/FlyWheel/FwAModel4/FWMath&ErrModel/Subsystem2/If Action Subsystem1 ==
  In1 : Inport
  Action Port : ActionPort  ActionType=else
  Out1 : Outport
  wires:
  In1/1 -> Out1/1

== system GS_model/Subsystem2/Subsystem/Actuator/FlyWheel/FwAModel4/FWMath&ErrModel/Subsystem2/Triggered Subsystem1 ==
  In1 : Inport
  Enable : EnablePort
  Out1 : Outport  InitialOutput=0
  wires:
  In1/1 -> Out1/1

== system GS_model/Subsystem2/Subsystem/Actuator/FlyWheel/FwAModel4/FWMath&ErrModel/Subsystem2/Triggered Subsystem2 ==
  In1 : Inport
  Enable : EnablePort
  Out1 : Outport  InitialOutput=0
  wires:
  In1/1 -> Out1/1

== system GS_model/Subsystem2/Subsystem/Actuator/FlyWheel/FwAModel4/FWMath&ErrModel/Subsystem4/If Action Subsystem ==
  In1 : Inport
  Action Port : ActionPort  ActionType=then
  Out1 : Outport
  wires:
  In1/1 -> Out1/1

== system GS_model/Subsystem2/Subsystem/Actuator/FlyWheel/FwAModel4/FWMath&ErrModel/Subsystem4/If Action Subsystem1 ==
  In1 : Inport
  Action Port : ActionPort  ActionType=else
  Out1 : Outport
  wires:
  In1/1 -> Out1/1

== system GS_model/Subsystem2/Subsystem/Actuator/FlyWheel/FwAModel4/FWMath&ErrModel/Subsystem4/Triggered Subsystem1 ==
  In1 : Inport
  Enable : EnablePort
  Out1 : Outport  InitialOutput=0
  wires:
  In1/1 -> Out1/1

== system GS_model/Subsystem2/Subsystem/Actuator/FlyWheel/FwAModel5/FWDataSourceChoice/DelayModel/delay1 ==
  In1 : Inport
  In2 : Inport  Port=2
  Delay : Delay  DelayLength=floor(T_Ctrl/T_Simu)
  Delay1 : Delay  DelayLength=2*floor(T_Ctrl/T_Simu)
  Delay2 : Delay  DelayLength=3*floor(T_Ctrl/T_Simu)
  Delay3 : Delay  DelayLength=4*floor(T_Ctrl/T_Simu)
  Multiport Switch : MultiPortSwitch  Inputs=5  SaturateOnIntegerOverflow=on
  Out1 : Outport
  wires:
  Delay1/1 -> Multiport Switch/4
  Delay2/1 -> Multiport Switch/5
  Delay3/1 -> Multiport Switch/6
  In1/1 -> Multiport Switch/1
  Multiport Switch/1 -> Out1/1
  In2/1 -> Multiport Switch/2, Delay1/1, Delay2/1, Delay3/1, Delay/1
  Delay/1 -> Multiport Switch/3

== system GS_model/Subsystem2/Subsystem/Actuator/FlyWheel/FwAModel5/FWDataSourceChoice/DelayModel/delay2 ==
  In1 : Inport
  In2 : Inport  Port=2
  Delay : Delay  DelayLength=floor(T_Ctrl/T_Simu)
  Delay1 : Delay  DelayLength=2*floor(T_Ctrl/T_Simu)
  Delay2 : Delay  DelayLength=3*floor(T_Ctrl/T_Simu)
  Delay3 : Delay  DelayLength=4*floor(T_Ctrl/T_Simu)
  Multiport Switch : MultiPortSwitch  Inputs=5  SaturateOnIntegerOverflow=on
  Out1 : Outport
  wires:
  Delay/1 -> Multiport Switch/3
  In2/1 -> Delay/1, Delay3/1, Delay2/1, Delay1/1, Multiport Switch/2
  Multiport Switch/1 -> Out1/1
  In1/1 -> Multiport Switch/1
  Delay3/1 -> Multiport Switch/6
  Delay2/1 -> Multiport Switch/5
  Delay1/1 -> Multiport Switch/4

== system GS_model/Subsystem2/Subsystem/Actuator/FlyWheel/FwAModel5/FWDataSourceChoice/DelayModel/delay3 ==
  In1 : Inport
  In2 : Inport  Port=2
  Delay : Delay  DelayLength=floor(T_Ctrl/T_Simu)
  Delay1 : Delay  DelayLength=2*floor(T_Ctrl/T_Simu)
  Delay2 : Delay  DelayLength=3*floor(T_Ctrl/T_Simu)
  Delay3 : Delay  DelayLength=4*floor(T_Ctrl/T_Simu)
  Multiport Switch : MultiPortSwitch  Inputs=5  SaturateOnIntegerOverflow=on
  Out1 : Outport
  wires:
  Delay1/1 -> Multiport Switch/4
  Delay2/1 -> Multiport Switch/5
  Delay3/1 -> Multiport Switch/6
  In1/1 -> Multiport Switch/1
  Multiport Switch/1 -> Out1/1
  In2/1 -> Multiport Switch/2, Delay1/1, Delay2/1, Delay3/1, Delay/1
  Delay/1 -> Multiport Switch/3

== system GS_model/Subsystem2/Subsystem/Actuator/FlyWheel/FwAModel5/FWMath&ErrModel/Subsystem1/If Action Subsystem ==
  In1 : Inport
  Action Port : ActionPort  ActionType=then
  Out1 : Outport
  wires:
  In1/1 -> Out1/1

== system GS_model/Subsystem2/Subsystem/Actuator/FlyWheel/FwAModel5/FWMath&ErrModel/Subsystem1/If Action Subsystem1 ==
  In1 : Inport
  Action Port : ActionPort  ActionType=else
  Out1 : Outport
  wires:
  In1/1 -> Out1/1

== system GS_model/Subsystem2/Subsystem/Actuator/FlyWheel/FwAModel5/FWMath&ErrModel/Subsystem1/Triggered Subsystem1 ==
  In1 : Inport
  Enable : EnablePort
  Out1 : Outport  InitialOutput=0
  wires:
  In1/1 -> Out1/1

== system GS_model/Subsystem2/Subsystem/Actuator/FlyWheel/FwAModel5/FWMath&ErrModel/Subsystem1/Triggered Subsystem2 ==
  In1 : Inport
  Enable : EnablePort
  Out1 : Outport  InitialOutput=0
  wires:
  In1/1 -> Out1/1

== system GS_model/Subsystem2/Subsystem/Actuator/FlyWheel/FwAModel5/FWMath&ErrModel/Subsystem2/If Action Subsystem ==
  In1 : Inport
  Action Port : ActionPort  ActionType=then
  Out1 : Outport
  wires:
  In1/1 -> Out1/1

== system GS_model/Subsystem2/Subsystem/Actuator/FlyWheel/FwAModel5/FWMath&ErrModel/Subsystem2/If Action Subsystem1 ==
  In1 : Inport
  Action Port : ActionPort  ActionType=else
  Out1 : Outport
  wires:
  In1/1 -> Out1/1

== system GS_model/Subsystem2/Subsystem/Actuator/FlyWheel/FwAModel5/FWMath&ErrModel/Subsystem2/Triggered Subsystem1 ==
  In1 : Inport
  Enable : EnablePort
  Out1 : Outport  InitialOutput=0
  wires:
  In1/1 -> Out1/1

== system GS_model/Subsystem2/Subsystem/Actuator/FlyWheel/FwAModel5/FWMath&ErrModel/Subsystem2/Triggered Subsystem2 ==
  In1 : Inport
  Enable : EnablePort
  Out1 : Outport  InitialOutput=0
  wires:
  In1/1 -> Out1/1

== system GS_model/Subsystem2/Subsystem/Actuator/FlyWheel/FwAModel5/FWMath&ErrModel/Subsystem4/If Action Subsystem ==
  In1 : Inport
  Action Port : ActionPort  ActionType=then
  Out1 : Outport
  wires:
  In1/1 -> Out1/1

== system GS_model/Subsystem2/Subsystem/Actuator/FlyWheel/FwAModel5/FWMath&ErrModel/Subsystem4/If Action Subsystem1 ==
  In1 : Inport
  Action Port : ActionPort  ActionType=else
  Out1 : Outport
  wires:
  In1/1 -> Out1/1

== system GS_model/Subsystem2/Subsystem/Actuator/FlyWheel/FwAModel5/FWMath&ErrModel/Subsystem4/Triggered Subsystem1 ==
  In1 : Inport
  Enable : EnablePort
  Out1 : Outport  InitialOutput=0
  wires:
  In1/1 -> Out1/1

== system GS_model/Subsystem2/Subsystem/Actuator/FlyWheel/FwAModel6/FWDataSourceChoice/DelayModel/delay1 ==
  In1 : Inport
  In2 : Inport  Port=2
  Delay : Delay  DelayLength=floor(T_Ctrl/T_Simu)
  Delay1 : Delay  DelayLength=2*floor(T_Ctrl/T_Simu)
  Delay2 : Delay  DelayLength=3*floor(T_Ctrl/T_Simu)
  Delay3 : Delay  DelayLength=4*floor(T_Ctrl/T_Simu)
  Multiport Switch : MultiPortSwitch  Inputs=5  SaturateOnIntegerOverflow=on
  Out1 : Outport
  wires:
  Delay/1 -> Multiport Switch/3
  In2/1 -> Delay/1, Delay3/1, Delay2/1, Delay1/1, Multiport Switch/2
  Multiport Switch/1 -> Out1/1
  In1/1 -> Multiport Switch/1
  Delay3/1 -> Multiport Switch/6
  Delay2/1 -> Multiport Switch/5
  Delay1/1 -> Multiport Switch/4

== system GS_model/Subsystem2/Subsystem/Actuator/FlyWheel/FwAModel6/FWDataSourceChoice/DelayModel/delay2 ==
  In1 : Inport
  In2 : Inport  Port=2
  Delay : Delay  DelayLength=floor(T_Ctrl/T_Simu)
  Delay1 : Delay  DelayLength=2*floor(T_Ctrl/T_Simu)
  Delay2 : Delay  DelayLength=3*floor(T_Ctrl/T_Simu)
  Delay3 : Delay  DelayLength=4*floor(T_Ctrl/T_Simu)
  Multiport Switch : MultiPortSwitch  Inputs=5  SaturateOnIntegerOverflow=on
  Out1 : Outport
  wires:
  Delay1/1 -> Multiport Switch/4
  Delay2/1 -> Multiport Switch/5
  Delay3/1 -> Multiport Switch/6
  In1/1 -> Multiport Switch/1
  Multiport Switch/1 -> Out1/1
  In2/1 -> Multiport Switch/2, Delay1/1, Delay2/1, Delay3/1, Delay/1
  Delay/1 -> Multiport Switch/3

== system GS_model/Subsystem2/Subsystem/Actuator/FlyWheel/FwAModel6/FWDataSourceChoice/DelayModel/delay3 ==
  In1 : Inport
  In2 : Inport  Port=2
  Delay : Delay  DelayLength=floor(T_Ctrl/T_Simu)
  Delay1 : Delay  DelayLength=2*floor(T_Ctrl/T_Simu)
  Delay2 : Delay  DelayLength=3*floor(T_Ctrl/T_Simu)
  Delay3 : Delay  DelayLength=4*floor(T_Ctrl/T_Simu)
  Multiport Switch : MultiPortSwitch  Inputs=5  SaturateOnIntegerOverflow=on
  Out1 : Outport
  wires:
  Delay/1 -> Multiport Switch/3
  In2/1 -> Delay/1, Delay3/1, Delay2/1, Delay1/1, Multiport Switch/2
  Multiport Switch/1 -> Out1/1
  In1/1 -> Multiport Switch/1
  Delay3/1 -> Multiport Switch/6
  Delay2/1 -> Multiport Switch/5
  Delay1/1 -> Multiport Switch/4

== system GS_model/Subsystem2/Subsystem/Actuator/FlyWheel/FwAModel6/FWMath&ErrModel/Subsystem1/If Action Subsystem ==
  In1 : Inport
  Action Port : ActionPort  ActionType=then
  Out1 : Outport
  wires:
  In1/1 -> Out1/1

== system GS_model/Subsystem2/Subsystem/Actuator/FlyWheel/FwAModel6/FWMath&ErrModel/Subsystem1/If Action Subsystem1 ==
  In1 : Inport
  Action Port : ActionPort  ActionType=else
  Out1 : Outport
  wires:
  In1/1 -> Out1/1

== system GS_model/Subsystem2/Subsystem/Actuator/FlyWheel/FwAModel6/FWMath&ErrModel/Subsystem1/Triggered Subsystem1 ==
  In1 : Inport
  Enable : EnablePort
  Out1 : Outport  InitialOutput=0
  wires:
  In1/1 -> Out1/1

== system GS_model/Subsystem2/Subsystem/Actuator/FlyWheel/FwAModel6/FWMath&ErrModel/Subsystem1/Triggered Subsystem2 ==
  In1 : Inport
  Enable : EnablePort
  Out1 : Outport  InitialOutput=0
  wires:
  In1/1 -> Out1/1

== system GS_model/Subsystem2/Subsystem/Actuator/FlyWheel/FwAModel6/FWMath&ErrModel/Subsystem2/If Action Subsystem ==
  In1 : Inport
  Action Port : ActionPort  ActionType=then
  Out1 : Outport
  wires:
  In1/1 -> Out1/1

== system GS_model/Subsystem2/Subsystem/Actuator/FlyWheel/FwAModel6/FWMath&ErrModel/Subsystem2/If Action Subsystem1 ==
  In1 : Inport
  Action Port : ActionPort  ActionType=else
  Out1 : Outport
  wires:
  In1/1 -> Out1/1

== system GS_model/Subsystem2/Subsystem/Actuator/FlyWheel/FwAModel6/FWMath&ErrModel/Subsystem2/Triggered Subsystem1 ==
  In1 : Inport
  Enable : EnablePort
  Out1 : Outport  InitialOutput=0
  wires:
  In1/1 -> Out1/1

== system GS_model/Subsystem2/Subsystem/Actuator/FlyWheel/FwAModel6/FWMath&ErrModel/Subsystem2/Triggered Subsystem2 ==
  In1 : Inport
  Enable : EnablePort
  Out1 : Outport  InitialOutput=0
  wires:
  In1/1 -> Out1/1

== system GS_model/Subsystem2/Subsystem/Actuator/FlyWheel/FwAModel6/FWMath&ErrModel/Subsystem4/If Action Subsystem ==
  In1 : Inport
  Action Port : ActionPort  ActionType=then
  Out1 : Outport
  wires:
  In1/1 -> Out1/1

== system GS_model/Subsystem2/Subsystem/Actuator/FlyWheel/FwAModel6/FWMath&ErrModel/Subsystem4/If Action Subsystem1 ==
  In1 : Inport
  Action Port : ActionPort  ActionType=else
  Out1 : Outport
  wires:
  In1/1 -> Out1/1

== system GS_model/Subsystem2/Subsystem/Actuator/FlyWheel/FwAModel6/FWMath&ErrModel/Subsystem4/Triggered Subsystem1 ==
  In1 : Inport
  Enable : EnablePort
  Out1 : Outport  InitialOutput=0
  wires:
  In1/1 -> Out1/1

== system GS_model/Subsystem2/Subsystem/Actuator/Magnetorquer/Mt_MathModel/MtA1/Mag_CmdCal/55//AA to +//- ==
  note: 55H:正向
      | AAH:负向
  In1 : Inport
  Add1 : Sum  Inputs=|++
  Cast To Double : DataTypeConversion  OutDataTypeStr=double
  Cast To Double2 : DataTypeConversion  OutDataTypeStr=double
  Compare To Constant : simulink/Logic and Bit Operations/Compare To Constant  relop===  const=85  OutDataTypeStr=boolean
  Compare To Constant1 : simulink/Logic and Bit Operations/Compare To Constant  relop===  const=170  OutDataTypeStr=boolean
  Constant1 : Constant  Value=-1
  Constant20 : Constant
  Product2 : Product  SaturateOnIntegerOverflow=on  OutDataTypeStr=Inherit: Same as first input
  Product6 : Product  SaturateOnIntegerOverflow=on  OutDataTypeStr=Inherit: Same as first input
  Out1 : Outport
  wires:
  Product6/1 -> Add1/1
  In1/1 -> Compare To Constant/1, Compare To Constant1/1
  Compare To Constant/1 -> Cast To Double/1
  Compare To Constant1/1 -> Cast To Double2/1
  Add1/1 -> Out1/1
  Cast To Double/1 -> Product6/2
  Constant20/1 -> Product6/1
  Product2/1 -> Add1/2
  Cast To Double2/1 -> Product2/1
  Constant1/1 -> Product2/2

== system GS_model/Subsystem2/Subsystem/Actuator/Magnetorquer/Mt_MathModel/MtA1/Mag_CmdCal/>=<0 to 012 ==
  note: 1--正向
  note: 0
  note: 2--负向
  In1 : Inport
  Add1 : Sum  Inputs=+++
  Cast To Double : DataTypeConversion  OutDataTypeStr=double
  Cast To Double1 : DataTypeConversion  OutDataTypeStr=double
  Cast To Double2 : DataTypeConversion  OutDataTypeStr=double
  Compare To Zero : simulink/Logic and Bit Operations/Compare To Zero  relop=<  OutDataTypeStr=boolean
  Compare To Zero1 : simulink/Logic and Bit Operations/Compare To Zero  relop===  OutDataTypeStr=uint8
  Compare To Zero2 : simulink/Logic and Bit Operations/Compare To Zero  relop=>  OutDataTypeStr=boolean
  Constant1 : Constant
  Constant2 : Constant  Value=0
  Constant20 : Constant  Value=2
  Product1 : Product  SaturateOnIntegerOverflow=on  OutDataTypeStr=Inherit: Same as first input
  Product2 : Product  SaturateOnIntegerOverflow=on  OutDataTypeStr=Inherit: Same as first input
  Product6 : Product  SaturateOnIntegerOverflow=on  OutDataTypeStr=Inherit: Same as first input
  Out1 : Outport
  wires:
  Product1/1 -> Add1/2
  Product6/1 -> Add1/1
  Compare To Zero1/1 -> Cast To Double1/1
  Constant2/1 -> Product1/1
  In1/1 -> Compare To Zero2/1, Compare To Zero1/1, Compare To Zero/1
  Compare To Zero/1 -> Cast To Double/1
  Compare To Zero2/1 -> Cast To Double2/1
  Add1/1 -> Out1/1
  Cast To Double/1 -> Product6/2
  Cast To Double1/1 -> Product1/2
  Constant20/1 -> Product6/1
  Constant1/1 -> Product2/1
  Cast To Double2/1 -> Product2/2
  Product2/1 -> Add1/3

== system GS_model/Subsystem2/Subsystem/Actuator/Magnetorquer/Mt_MathModel/MtA2/Mag_CmdCal/55//AA to +//- ==
  note: 55H:正向
      | AAH:负向
  In1 : Inport
  Add1 : Sum  Inputs=|++
  Cast To Double : DataTypeConversion  OutDataTypeStr=double
  Cast To Double2 : DataTypeConversion  OutDataTypeStr=double
  Compare To Constant : simulink/Logic and Bit Operations/Compare To Constant  relop===  const=85  OutDataTypeStr=boolean
  Compare To Constant1 : simulink/Logic and Bit Operations/Compare To Constant  relop===  const=170  OutDataTypeStr=boolean
  Constant1 : Constant  Value=-1
  Constant20 : Constant
  Product2 : Product  SaturateOnIntegerOverflow=on  OutDataTypeStr=Inherit: Same as first input
  Product6 : Product  SaturateOnIntegerOverflow=on  OutDataTypeStr=Inherit: Same as first input
  Out1 : Outport
  wires:
  Constant1/1 -> Product2/2
  Cast To Double2/1 -> Product2/1
  Product2/1 -> Add1/2
  Constant20/1 -> Product6/1
  Cast To Double/1 -> Product6/2
  Add1/1 -> Out1/1
  Compare To Constant1/1 -> Cast To Double2/1
  Compare To Constant/1 -> Cast To Double/1
  In1/1 -> Compare To Constant1/1, Compare To Constant/1
  Product6/1 -> Add1/1

== system GS_model/Subsystem2/Subsystem/Actuator/Magnetorquer/Mt_MathModel/MtA2/Mag_CmdCal/>=<0 to 012 ==
  note: 2--负向
  note: 0
  note: 1--正向
  In1 : Inport
  Add1 : Sum  Inputs=+++
  Cast To Double : DataTypeConversion  OutDataTypeStr=double
  Cast To Double1 : DataTypeConversion  OutDataTypeStr=double
  Cast To Double2 : DataTypeConversion  OutDataTypeStr=double
  Compare To Zero : simulink/Logic and Bit Operations/Compare To Zero  relop=<  OutDataTypeStr=boolean
  Compare To Zero1 : simulink/Logic and Bit Operations/Compare To Zero  relop===  OutDataTypeStr=uint8
  Compare To Zero2 : simulink/Logic and Bit Operations/Compare To Zero  relop=>  OutDataTypeStr=boolean
  Constant1 : Constant
  Constant2 : Constant  Value=0
  Constant20 : Constant  Value=2
  Product1 : Product  SaturateOnIntegerOverflow=on  OutDataTypeStr=Inherit: Same as first input
  Product2 : Product  SaturateOnIntegerOverflow=on  OutDataTypeStr=Inherit: Same as first input
  Product6 : Product  SaturateOnIntegerOverflow=on  OutDataTypeStr=Inherit: Same as first input
  Out1 : Outport
  wires:
  Product2/1 -> Add1/3
  Cast To Double2/1 -> Product2/2
  Constant1/1 -> Product2/1
  Constant20/1 -> Product6/1
  Cast To Double1/1 -> Product1/2
  Cast To Double/1 -> Product6/2
  Add1/1 -> Out1/1
  Compare To Zero2/1 -> Cast To Double2/1
  Compare To Zero/1 -> Cast To Double/1
  In1/1 -> Compare To Zero/1, Compare To Zero1/1, Compare To Zero2/1
  Constant2/1 -> Product1/1
  Compare To Zero1/1 -> Cast To Double1/1
  Product6/1 -> Add1/1
  Product1/1 -> Add1/2

== system GS_model/Subsystem2/Subsystem/Actuator/Magnetorquer/Mt_MathModel/MtA3/Mag_CmdCal/55//AA to +//- ==
  note: 55H:正向
      | AAH:负向
  In1 : Inport
  Add1 : Sum  Inputs=|++
  Cast To Double : DataTypeConversion  OutDataTypeStr=double
  Cast To Double2 : DataTypeConversion  OutDataTypeStr=double
  Compare To Constant : simulink/Logic and Bit Operations/Compare To Constant  relop===  const=85  OutDataTypeStr=boolean
  Compare To Constant1 : simulink/Logic and Bit Operations/Compare To Constant  relop===  const=170  OutDataTypeStr=boolean
  Constant1 : Constant  Value=-1
  Constant20 : Constant
  Product2 : Product  SaturateOnIntegerOverflow=on  OutDataTypeStr=Inherit: Same as first input
  Product6 : Product  SaturateOnIntegerOverflow=on  OutDataTypeStr=Inherit: Same as first input
  Out1 : Outport
  wires:
  Product6/1 -> Add1/1
  In1/1 -> Compare To Constant/1, Compare To Constant1/1
  Compare To Constant/1 -> Cast To Double/1
  Compare To Constant1/1 -> Cast To Double2/1
  Add1/1 -> Out1/1
  Cast To Double/1 -> Product6/2
  Constant20/1 -> Product6/1
  Product2/1 -> Add1/2
  Cast To Double2/1 -> Product2/1
  Constant1/1 -> Product2/2
